simulink model "rtwdemo_targetsettings"  (Simulink 6.0)
settings: Solver=FixedStepDiscrete  StartTime=0.0  StopTime=1  FixedStep=1  RelTol=1e-3
libraries: rtwdemowidgets x3
settings Model: Creator=The MathWorks Inc.  LastModifiedBy=batserve  ExtModeTrigMode=oneshot  ExtModeArmWhenConnect=off  ExtModeAutoUpdateStatusClock=off
settings DataIOCC: LimitDataPoints=off  SaveOutput=off  SaveTime=off  SignalLoggingName=logsOut
settings OptimizationCC: InlineParams=on  EnforceIntegerDowncast=off  StateBitsets=on  DataBitsets=on  UseTempVars=on
settings DebuggingCC: CheckExecutionContextPreStartOutputMsg=on  CheckExecutionContextRuntimeOutputMsg=on  SolverPrmCheckMsg=none  IntegerOverflowMsg=none
settings HardwareCC: TargetHWDeviceType=32-bit Generic
settings ModelReferenceCC: UpdateModelReferenceTargets=IfOutOfDate
settings RTWCC: GenerateReport=on  RTWVerbose=off  ProcessScript=grt_make_rtw_hook  LaunchReport=on
settings CodeAppCC: ForceParamTrailComments=on
settings GRTTargetCC: MatFileLogging=off

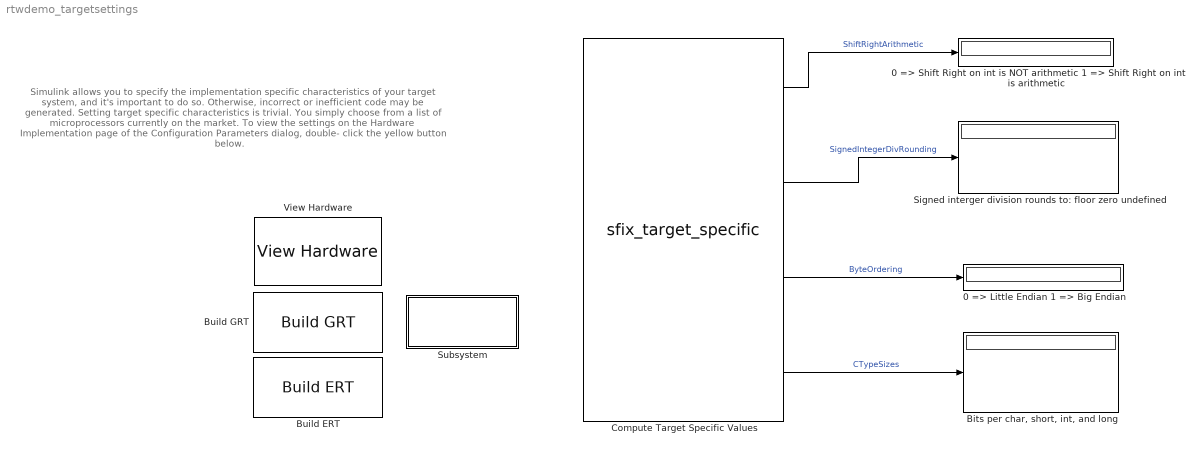
== system rtwdemo_targetsettings ==
  note: Simulink allows you to specify the implementation
      | specific characteristics of your target system, and
      | it's important to do so.  Otherwise, incorrect or
      | inefficient code may be generated.
      |
      | Setting target specific characteristics is trivial.
      | You simply choose from a list of microprocessors
      | currently on the market.
      |
      | To view the settings on the Hardware Implementation
      | page of the Configuration Parameters dialog, double-
      | click the yellow button below.
  "0 => Little Endian 1 => Big Endian   " : Display
  "0 => Shift Right on int is NOT arithmetic 1 => Shift Right on int is arithmetic    " : Display
  "Bits per char, short, int, and long" : Display
  Build ERT : rtwdemowidgets/Build ERT  attrib_overrides={}
  Build GRT : rtwdemowidgets/Build GRT  attrib_overrides={}
  Compute Target Specific Values : S-Function  FunctionName=sfix_target_specific
      mask Type: Fixed-Point Target Specific
      mask Description: Used to get information about a fixed point target compiler/processor.
      mask Help: web(fpbhelp);
      mask Display:
      | port_label('output',1,'Shift Right on int is arithmetic' );
      | port_label('output',2,'Signed integer division rounding' );
      | port_label('output',3,'Byte ordering' );
      | port_label('output',4,'Bits per char, short, int, long' );
  Signed interger division rounds to: floor zero undefined : Display
  Subsystem : Subsystem  PropExecContextAcrossSSBoundary=on
      mask Display: disp(['My microprocessor\nis not listed ..','.        '])
  View Hardware : rtwdemowidgets/View Hardware
  wires:
  Compute Target Specific Values/3 -> "0 => Little Endian 1 => Big Endian   "/1  "ByteOrdering"
  Compute Target Specific Values/4 -> "Bits per char, short, int, and long"/1  "CTypeSizes"
  Compute Target Specific Values/1 -> "0 => Shift Right on int is NOT arithmetic 1 => Shift Right on int is arithmetic    "/1  "ShiftRightArithmetic"
  Compute Target Specific Values/2 -> Signed interger division rounds to: floor zero undefined/1  "SignedIntegerDivRounding"

== system rtwdemo_targetsettings/Subsystem ==
  note: If your system is not listed and you are not certain of its values, use the code generated
      | by this model to compute the necessary C compiler and target hardware settings.
      |
      | If you use a cross-development system that includes a source level debugger, first
      | configure the model for your intended target. Then, generate code and build an executable
      | using your target development system.  Download the executable to the target and set
      | breakpoints at the model output code for each of the outports of the model.  Run a
      | debugging session and observe the behavior of the code as it executes on the target.
      | As you step through the code the values for the various characteristics are computed.
      |
      | If your target development system does not support source level debugging, you may have to
      | generate code and add printf statements or other code that enables you to obtain the
      | results.
      |
      | Once you've obtained your target settings, enter them into the Hardware Implementation
      | page via a 'Custom' device type.
